simulink model "CoppeliaSimulink"  (R2021a)
settings: Solver=VariableStepAuto  StartTime=0.0  StopTime=inf  RelTol=1e-3
settings Model: Creator=josef  LastModifiedBy=josef

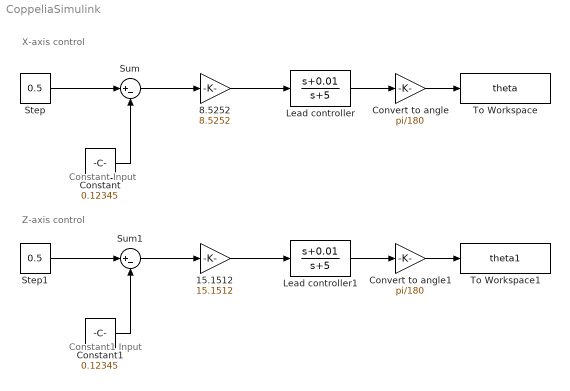
== system CoppeliaSimulink ==
  note: X-axis control
  note: Constant Input
  note: Constant1 Input
  note: Z-axis control
  15.1512 : Gain  Gain=15.1512
  8.5252 : Gain  Gain=8.5252
  Constant : Constant  Value=0.12345
  Constant1 : Constant  Value=0.12345
  Convert to angle : Gain  Gain=pi/180
  Convert to angle1 : Gain  Gain=pi/180
  Lead controller : TransferFcn  Numerator=[1 0.01]  Denominator=[1 5]
  Lead controller1 : TransferFcn  Numerator=[1 0.01]  Denominator=[1 5]
  Step : Constant  Value=0.5
  Step1 : Constant  Value=0.5
  Sum : Sum  Inputs=|+-
  Sum1 : Sum  Inputs=|+-
  To Workspace : ToWorkspace  VariableName=theta  SaveFormat=Timeseries  SampleTime=-1
  To Workspace1 : ToWorkspace  VariableName=theta1  SaveFormat=Timeseries  SampleTime=-1
  wires:
  Step/1 -> Sum/1
  Sum/1 -> 8.5252/1
  8.5252/1 -> Lead controller/1
  Constant/1 -> Sum/2
  Lead controller/1 -> Convert to angle/1
  Convert to angle/1 -> To Workspace/1
  Constant1/1 -> Sum1/2
  Lead controller1/1 -> Convert to angle1/1
  Convert to angle1/1 -> To Workspace1/1
  15.1512/1 -> Lead controller1/1
  Sum1/1 -> 15.1512/1
  Step1/1 -> Sum1/1
